simulink model "DC_MOTOR"  (R2016a)
settings: Solver=VariableStepAuto  StartTime=0.0  StopTime=10.0  RelTol=1e-3
libraries: fuzblock x1, simulink_extras x1
settings Model: Creator=User  LastModifiedBy=User

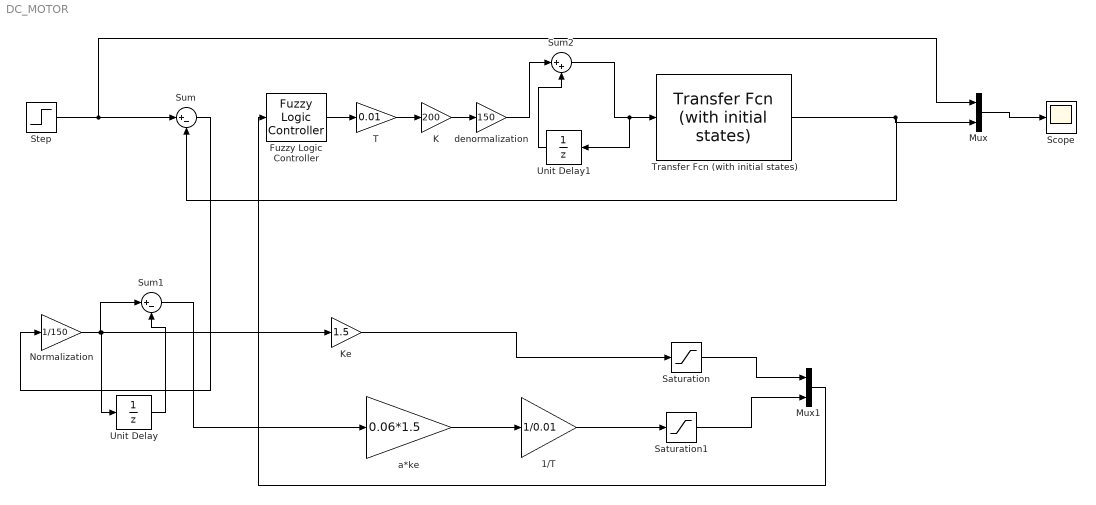
== system DC_MOTOR ==
  1/T : Gain  Gain=1/0.01
  Fuzzy Logic Controller : fuzblock/Fuzzy Logic  Controller  fis='DC_MOTOR.fis'
  K : Gain  Gain=200
  Ke : Gain  Gain=1.5
  Mux : Mux  Inputs=2
  Mux1 : Mux  Inputs=2
  Normalization : Gain  Gain=1/150
  Saturation : Saturate
  Saturation1 : Saturate
  Scope : Scope
  Step : Step  After=150  SampleTime=0
  Sum : Sum  Inputs=|+-
  Sum1 : Sum  Inputs=|+-
  Sum2 : Sum  Inputs=|++
  T : Gain  Gain=0.01
  Transfer Fcn (with initial states) : simulink_extras/Additional Linear/Transfer Fcn (with initial states)  N=[12 225]  D=[1 24 225]  X0=.5
  Unit Delay : UnitDelay
  Unit Delay1 : UnitDelay
  a*ke : Gain  Gain=0.06*1.5
  denormalization : Gain  Gain=150
  wires:
  Step/1 -> Mux/1, Sum/1
  a*ke/1 -> 1/T/1
  Mux1/1 -> Fuzzy Logic Controller/1
  Fuzzy Logic Controller/1 -> T/1
  T/1 -> K/1
  K/1 -> denormalization/1
  Normalization/1 -> Ke/1, Unit Delay/1, Sum1/1
  Unit Delay/1 -> Sum1/2
  Sum1/1 -> a*ke/1
  denormalization/1 -> Sum2/1
  Sum2/1 -> Unit Delay1/1, Transfer Fcn (with initial states)/1
  Unit Delay1/1 -> Sum2/2
  Transfer Fcn (with initial states)/1 -> Mux/2, Sum/2
  Mux/1 -> Scope/1
  Ke/1 -> Saturation/1
  Saturation/1 -> Mux1/1
  1/T/1 -> Saturation1/1
  Saturation1/1 -> Mux1/2
  Sum/1 -> Normalization/1
